simulink model "model"  (R2019b)
settings: Solver=VariableStepAuto  StartTime=0.0  StopTime=30  RelTol=1e-3
InitFcn:
  | parameters;
  | initialize;
undefined symbols (not defined in the file): drawVehicle, K, state_init, T, u0, x0
settings Model: Creator=louis  LastModifiedBy=louis
settings DataIOCC: ReturnWorkspaceOutputs=off

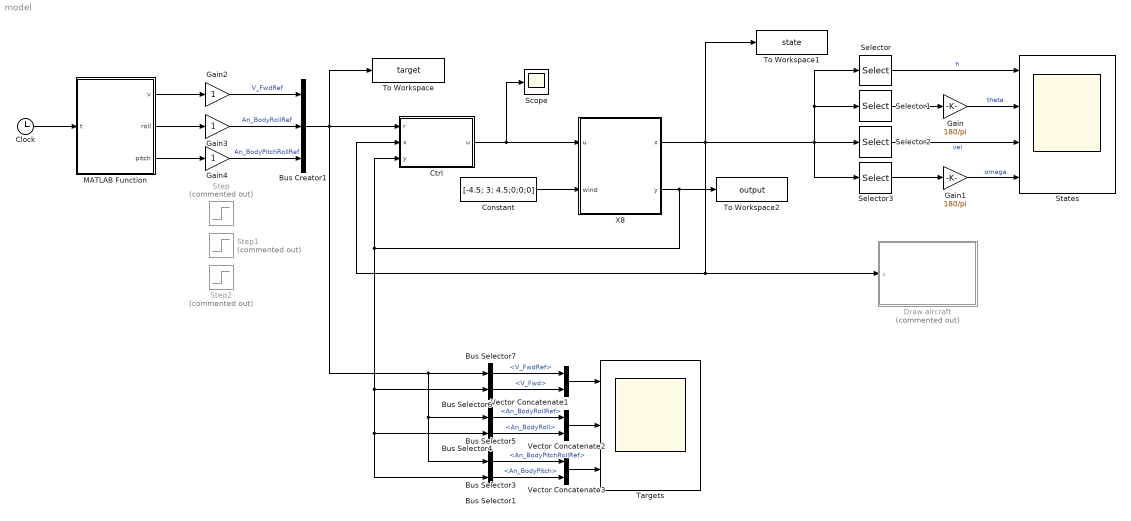
== system model ==
  Bus Creator1 : BusCreator  Inputs=3
  Bus Selector1 : BusSelector  OutputSignals=An_BodyPitch
  Bus Selector3 : BusSelector  OutputSignals=An_BodyPitchRollRef
  Bus Selector4 : BusSelector  OutputSignals=An_BodyRoll
  Bus Selector5 : BusSelector  OutputSignals=An_BodyRollRef
  Bus Selector6 : BusSelector  OutputSignals=V_Fwd
  Bus Selector7 : BusSelector  OutputSignals=V_FwdRef
  Clock : Clock
  Constant : Constant  Value=[-4.5; 3; 4.5;0;0;0]
  Ctrl : Subsystem
      mask init:
      | load('controller')
      mask Display: image(imread('kestrel.jpg'))
  Draw aircraft : Subsystem  Commented=on
      mask Display: image(imread('crazyflie.jpg'))
  Gain : Gain  Gain=180/pi
  Gain1 : Gain  Gain=180/pi
  Gain2 : Gain
  Gain3 : Gain
  Gain4 : Gain
  MATLAB Function : MATLAB Function  TreatAsAtomicUnit=on
  Scope : Scope
  Selector : Selector  IndexOptions=Index vector (dialog)  Indices=3  OutputSizes=1
  Selector1 : Selector  IndexOptions=Index vector (dialog)  Indices=4:6  OutputSizes=1
  Selector2 : Selector  IndexOptions=Index vector (dialog)  Indices=7:9  OutputSizes=1
  Selector3 : Selector  IndexOptions=Index vector (dialog)  Indices=10:12  OutputSizes=1
  States : Scope  NumInputPorts=4
  Step : Step  Commented=on  Before=18  After=20  SampleTime=0
  Step1 : Step  Commented=on  After=pi/180*10  SampleTime=0
  Step2 : Step  Commented=on  After=pi/180*10  SampleTime=0
  Targets : Scope  NumInputPorts=3
  To Workspace : ToWorkspace  VariableName=target  SaveFormat=Timeseries  SampleTime=-1
  To Workspace1 : ToWorkspace  VariableName=state  SaveFormat=Timeseries  SampleTime=-1
  To Workspace2 : ToWorkspace  VariableName=output  SaveFormat=Timeseries  SampleTime=-1
  Vector Concatenate1 : Concatenate
  Vector Concatenate2 : Concatenate
  Vector Concatenate3 : Concatenate
  X8 : Subsystem
  wires:
  Selector/1 -> States/1  "h"
  Selector1/1 -> Gain/1
  Selector2/1 -> States/3  "vel"
  Selector3/1 -> Gain1/1
  Gain/1 -> States/2  "theta"
  Gain1/1 -> States/4  "omega"
  Constant/1 -> X8/2(wind)
  X8/2(y) -> Ctrl/3(y), Bus Selector6/1, Bus Selector4/1, Bus Selector1/1, To Workspace2/1
  Ctrl/1(u) -> Scope/1, X8/1(u)
  X8/1(x) -> To Workspace1/1, Selector3/1, Selector/1, Selector1/1, Selector2/1, Draw aircraft/1(x), Ctrl/2(x)
  Bus Creator1/1 -> To Workspace/1, Bus Selector5/1, Bus Selector3/1, Bus Selector7/1, Ctrl/1(r)
  Vector Concatenate1/1 -> Targets/1
  Vector Concatenate2/1 -> Targets/2
  Vector Concatenate3/1 -> Targets/3
  Bus Selector1/1 -> Vector Concatenate3/2  "<An_BodyPitch>"
  Bus Selector3/1 -> Vector Concatenate3/1  "<An_BodyPitchRollRef>"
  Bus Selector4/1 -> Vector Concatenate2/2  "<An_BodyRoll>"
  Bus Selector5/1 -> Vector Concatenate2/1  "<An_BodyRollRef>"
  Bus Selector6/1 -> Vector Concatenate1/2  "<V_Fwd>"
  Bus Selector7/1 -> Vector Concatenate1/1  "<V_FwdRef>"
  Gain2/1 -> Bus Creator1/1  "V_FwdRef"
  Gain3/1 -> Bus Creator1/2  "An_BodyRollRef"
  Gain4/1 -> Bus Creator1/3  "An_BodyPitchRollRef"
  Clock/1 -> MATLAB Function/1(t)
  MATLAB Function/1(v) -> Gain2/1
  MATLAB Function/2(roll) -> Gain3/1
  MATLAB Function/3(pitch) -> Gain4/1

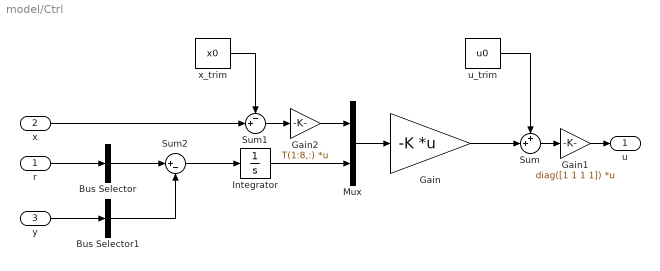
== system model/Ctrl ==
  r : Inport
  x : Inport  Port=2
  y : Inport  Port=3
  Bus Selector : BusSelector  OutputSignals=An_BodyRollRef,An_BodyPitchRollRef  OutputAsBus=on
  Bus Selector1 : BusSelector  OutputSignals=An_BodyRoll,An_BodyPitch  OutputAsBus=on
  Gain : Gain  Gain=-K  Multiplication=Matrix(K*u) (u vector)
  Gain1 : Gain  Gain=diag([1 1 1 1])  Multiplication=Matrix(K*u) (u vector)
  Gain2 : Gain  Gain=T(1:8,:)  Multiplication=Matrix(K*u) (u vector)
  Integrator : Integrator
  Mux : Mux  Inputs=2
  Sum : Sum  Inputs=++|
  Sum1 : Sum  Inputs=-+|
  Sum2 : Sum  Inputs=|+-
  u_trim : Constant  Value=u0
  x_trim : Constant  Value=x0
  u : Outport
  wires:
  Gain/1 -> Sum/2
  u_trim/1 -> Sum/1
  Sum/1 -> Gain1/1
  x_trim/1 -> Sum1/1
  Sum1/1 -> Gain2/1
  x/1 -> Sum1/2
  Bus Selector/1 -> Sum2/1
  Bus Selector1/1 -> Sum2/2
  Sum2/1 -> Integrator/1
  Mux/1 -> Gain/1
  Integrator/1 -> Mux/2
  Gain2/1 -> Mux/1
  Gain1/1 -> u/1
  r/1 -> Bus Selector/1
  y/1 -> Bus Selector1/1

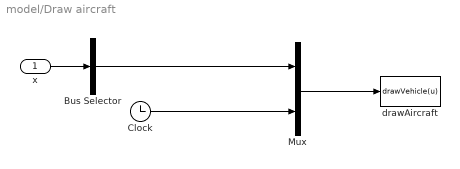
== system model/Draw aircraft ==
  x : Inport
  Bus Selector : BusSelector  OutputSignals=L_PosNorth,L_PosEast,L_PosH,V_Fwd,V_Lat,V_Vert,An_BodyRoll,An_BodyPitch,An_BodyYaw,W_RollRate,W_PitchRate,W_YawRate  OutputAsBus=on
  Clock : Clock
  Mux : Mux  Inputs=2
  drawAircraft : MATLABFcn  MATLABFcn=drawVehicle(u)  OutputDimensions=0  SampleTime=0.05
  wires:
  Clock/1 -> Mux/2
  Bus Selector/1 -> Mux/1
  Mux/1 -> drawAircraft/1
  x/1 -> Bus Selector/1

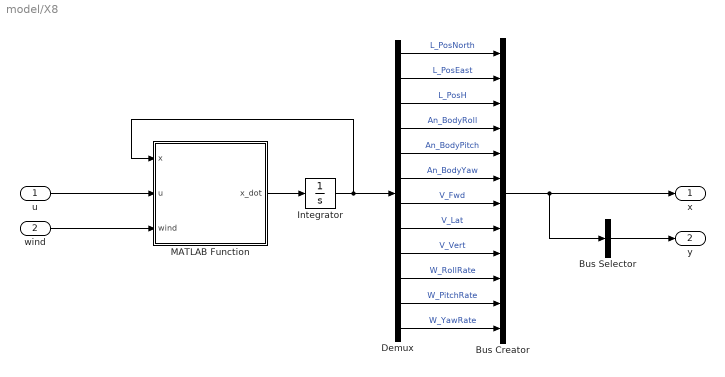
== system model/X8 ==
  u : Inport
  wind : Inport  Port=2
  Bus Creator : BusCreator  Inputs=12
  Bus Selector : BusSelector  OutputSignals=V_Fwd,An_BodyRoll,An_BodyPitch  OutputAsBus=on
  Demux : Demux  Outputs=12
  Integrator : Integrator  InitialCondition=state_init
  MATLAB Function : MATLAB Function  TreatAsAtomicUnit=on
  x : Outport
  y : Outport  Port=2
  wires:
  Integrator/1 -> MATLAB Function/1(x), Demux/1
  u/1 -> MATLAB Function/2(u)
  MATLAB Function/1(x_dot) -> Integrator/1
  wind/1 -> MATLAB Function/3(wind)
  Demux/1 -> Bus Creator/1  "L_PosNorth"
  Demux/2 -> Bus Creator/2  "L_PosEast"
  Demux/3 -> Bus Creator/3  "L_PosH"
  Demux/4 -> Bus Creator/4  "An_BodyRoll"
  Demux/5 -> Bus Creator/5  "An_BodyPitch"
  Demux/6 -> Bus Creator/6  "An_BodyYaw"
  Demux/7 -> Bus Creator/7  "V_Fwd"
  Demux/8 -> Bus Creator/8  "V_Lat"
  Demux/9 -> Bus Creator/9  "V_Vert"
  Demux/10 -> Bus Creator/10  "W_RollRate"
  Demux/11 -> Bus Creator/11  "W_PitchRate"
  Demux/12 -> Bus Creator/12  "W_YawRate"
  Bus Creator/1 -> Bus Selector/1, x/1
  Bus Selector/1 -> y/1

== matlab function model/MATLAB Function ==
  data: t input; v output; roll output; pitch output
function [v, roll, pitch] = target(t)

%% Velocity target
v = 18;

%% Roll angle target
if t < 5
    roll = 0;
elseif t < 10
    roll = -15;
elseif t < 15
    roll = 5;
elseif t < 20
    roll = -5;
elseif t < 25
    roll = 30;
else
    roll = 60;
end

roll = roll * pi/180;

%% Pitch angle
if t < 5
    pitch = 0;
elseif t < 10
    pitch = 10;
elseif t < 15
    pitch = -25;
elseif t < 20
    pitch = 5;
elseif t < 25
    pitch = -5;
else
    pitch = 20;
end

pitch = pitch * pi/180;

end

== matlab function model/X8/MATLAB Function ==
  data: x input; u input; x_dot output; wind input; P parameter
function x_dot = model(x,u,wind,P)

x_dot = dynamics(x,u,wind,P);

end
